simulink model "pend_on_cart"  (R2021a)
settings: Solver=VariableStepAuto  StartTime=0.0  StopTime=1  RelTol=1e-3
(part 1 of 3)
settings Model: Creator=onurc  LastModifiedBy=onurc

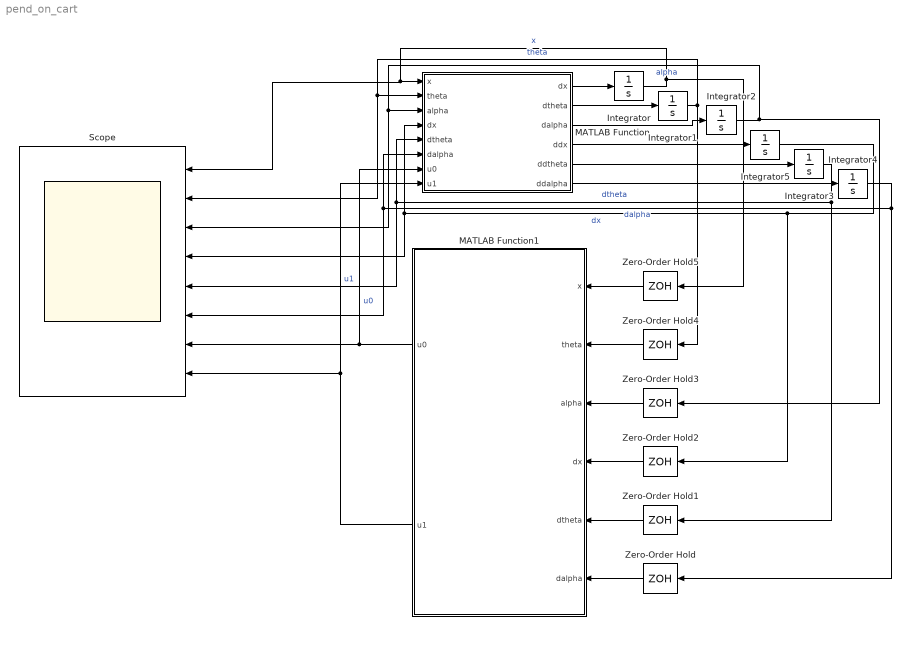
== system pend_on_cart ==
  Integrator : Integrator  InitialCondition=1
  Integrator{1..5} (5 alike) : Integrator
  MATLAB Function : MATLAB Function  TreatAsAtomicUnit=on
  MATLAB Function1 : MATLAB Function  TreatAsAtomicUnit=on
  Scope : Scope  NumInputPorts=8
  Zero-Order Hold{,1..5} (6 alike) : ZeroOrderHold  SampleTime=0.001
  wires:
  Integrator2/1 -> Zero-Order Hold3/1, Scope/3, MATLAB Function/3(alpha)  "alpha"
  MATLAB Function/1(dx) -> Integrator/1
  MATLAB Function/2(dtheta) -> Integrator1/1
  MATLAB Function/3(dalpha) -> Integrator2/1
  MATLAB Function/4(ddx) -> Integrator5/1
  MATLAB Function/5(ddtheta) -> Integrator3/1
  MATLAB Function/6(ddalpha) -> Integrator4/1
  Integrator/1 -> Zero-Order Hold5/1, Scope/1, MATLAB Function/1(x)  "x"
  Integrator1/1 -> Zero-Order Hold4/1, Scope/2, MATLAB Function/2(theta)  "theta"
  Integrator5/1 -> Zero-Order Hold2/1, MATLAB Function/4("dx "), Scope/4  "dx"
  Integrator3/1 -> Zero-Order Hold1/1, MATLAB Function/5("dtheta "), Scope/5  "dtheta"
  Integrator4/1 -> Zero-Order Hold/1, MATLAB Function/6("dalpha "), Scope/6  "dalpha"
  MATLAB Function1/1(u0) -> Scope/7, MATLAB Function/7(u0)  "u0"
  MATLAB Function1/2(u1) -> Scope/8, MATLAB Function/8(u1)  "u1"
  Zero-Order Hold5/1 -> MATLAB Function1/1(x)
  Zero-Order Hold/1 -> MATLAB Function1/6(dalpha)
  Zero-Order Hold1/1 -> MATLAB Function1/5(dtheta)
  Zero-Order Hold2/1 -> MATLAB Function1/4(dx)
  Zero-Order Hold3/1 -> MATLAB Function1/3(alpha)
  Zero-Order Hold4/1 -> MATLAB Function1/2(theta)
